simulink library "fdclib3"  (Simulink 2.09)
values from neighbouring files (symbols this model uses):
  GM1 = [cbar b    S    Ix   Iy   Iz   Jxy  Jxz  Jyz  m]    [modbuild.m]

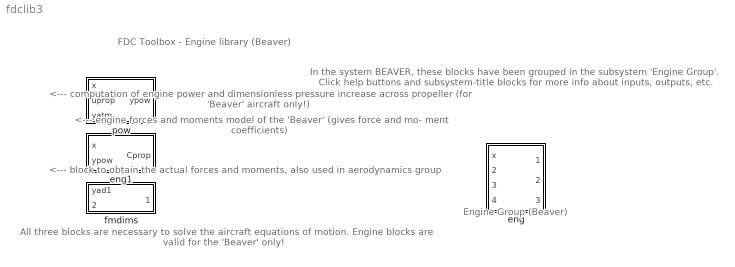
== system fdclib3 ==
  note: FDC Toolbox - Engine library (Beaver)
  note: All three blocks are necessary to solve the aircraft equations
      | of motion. Engine blocks are valid for the 'Beaver' only!
  note: Engine Group
      | (Beaver)
  note: In the system BEAVER, these blocks have
      | been grouped in the subsystem 'Engine Group'.
      | Click help buttons and subsystem-title blocks
      | for more info about inputs, outputs, etc.
  note: <--- block to obtain the actual
      |       forces and moments, also used
      | in aerodynamics group
  note: <--- engine forces and moments model
      | of the 'Beaver' (gives force and mo-
      | ment coefficients)
  note: <--- computation of engine power and
      | dimensionless pressure increase across
      | propeller (for 'Beaver' aircraft only!)
  eng : Subsystem
  eng1 : Subsystem
      mask Type: Engmod
      mask Description: Engine model for the DHC-2 'Beaver'
      mask Help: eval('fdchelp engmod')
      mask Display: disp('Engmod\n(Beaver)')
  fmdims : Subsystem  mask(FMdims){cbar=GM1(1), b=GM1(2), S=GM1(3)}
      mask prompts: cbar "Mean aerodynamic chord [m]:"; b "Wing span [m]:"; S "Wing surface [m^2]:"
      mask help:
      | Calculate forces and moments from
      | dimensionless coefficients.
      mask Help: eval('fdchelp fmdims')
      mask Display: disp('FMdims')
  pow : Subsystem
      mask Type: Power
      mask Description:
      | Engine power and dimensionless
      | pressure increase across propeller
      | (model for DHC-2 'Beaver')
      mask Help: eval('fdchelp power')
      mask Display: disp('Power\n(Beaver)')

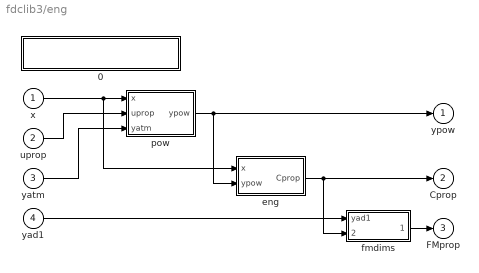
== system fdclib3/eng ==
  x : Inport  Port=1  PortWidth=-1  SampleTime=-1
  uprop : Inport  Port=2  PortWidth=-1  SampleTime=-1
  yatm : Inport  Port=3  PortWidth=-1  SampleTime=-1
  yad1 : Inport  Port=4  PortWidth=-1  SampleTime=-1
  0 : Subsystem
      settings: OpenFcn=fdchelp enggrp
      mask Display: disp('ENGINE GROUP (level 3)\nM.O. Rauw')
  eng : Subsystem
      mask Type: Engmod
      mask Description: Engine model for the DHC-2 'Beaver'
      mask Help: eval('fdchelp engmod')
      mask Display: disp('Engmod\n(Beaver)')
  fmdims : Subsystem  mask(FMdims){cbar=GM1(1), b=GM1(2), S=GM1(3)}
      mask prompts: cbar "Mean aerodynamic chord [m]:"; b "Wing span [m]:"; S "Wing surface [m^2]:"
      mask help:
      | Calculate forces and moments from
      | dimensionless coefficients.
      mask Help: eval('fdchelp fmdims')
      mask Display: disp('FMdims')
  pow : Subsystem
      mask Type: Power
      mask Description:
      | Engine power and dimensionless
      | pressure increase across propeller
      | (model for DHC-2 'Beaver')
      mask Help: eval('fdchelp power')
      mask Display: disp('Power\n(Beaver)')
  ypow : Outport  Port=1  InitialOutput=0
  Cprop : Outport  Port=2  InitialOutput=0
  FMprop : Outport  Port=3  InitialOutput=0
  wires:
  yatm/1 -> pow/3(yatm)
  x/1 -> eng/1(x), pow/1(x)
  yad1/1 -> fmdims/1(yad1)
  eng/1(Cprop) -> fmdims/2(Force / moment coefficients), Cprop/1
  fmdims/1(Forces and moments) -> FMprop/1
  uprop/1 -> pow/2(uprop)
  pow/1(ypow) -> eng/2(ypow), ypow/1

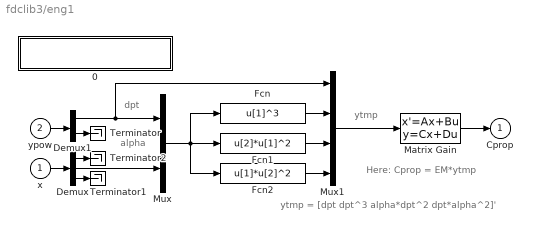
== system fdclib3/eng1 ==
  note: ytmp
  note: alpha
  note: dpt
  note: ytmp = [dpt dpt^3 alpha*dpt^2 dpt*alpha^2]'
  note: Here: Cprop = EM*ytmp
  x : Inport  Port=1  PortWidth=-1  SampleTime=-1
  ypow : Inport  Port=2  PortWidth=-1  SampleTime=-1
  0 : Subsystem
      settings: OpenFcn=fdchelp engmod
      mask Display: disp('ENGMOD\nM.O. Rauw, Dec. 1996')
  Demux : Demux  Outputs=[1 1 10]
  Demux1 : Demux  Outputs=2
  Fcn : Fcn  Expr=u[1]^3
  Fcn1 : Fcn  Expr=u[2]*u[1]^2
  Fcn2 : Fcn  Expr=u[1]*u[2]^2
  Matrix Gain : StateSpace  A=A  B=B  C=C  D=D  X0=0  mask(Matrix Gain){@1=EM}
      mask prompts: @1 "Gain matrix:"
      mask help: Matrix Gain
      mask init:
      | A = []; B = []; C = []; D = @1;
      mask Help: This block implements an matrix gain.\nThe matrix dimensions must be in accordance\nwith the dimension of the inputvector.
      mask Display: disp('y = A*u')
  Mux : Mux  Inputs=2
  Mux1 : Mux  Inputs=4
  Terminator : Terminator
  Terminator1 : Terminator
  Terminator2 : Terminator
  Cprop : Outport  Port=1  InitialOutput=0
  wires:
  Fcn2/1 -> Mux1/4
  Fcn1/1 -> Mux1/3
  Fcn/1 -> Mux1/2
  Demux1/1 -> Mux1/1, Mux/1
  Mux/1 -> Fcn2/1, Fcn/1, Fcn1/1
  Demux/2 -> Mux/2
  ypow/1 -> Demux1/1
  x/1 -> Demux/1
  Mux1/1 -> Matrix Gain/1
  Matrix Gain/1 -> Cprop/1
  Demux1/2 -> Terminator/1
  Demux/3 -> Terminator1/1
  Demux/1 -> Terminator2/1

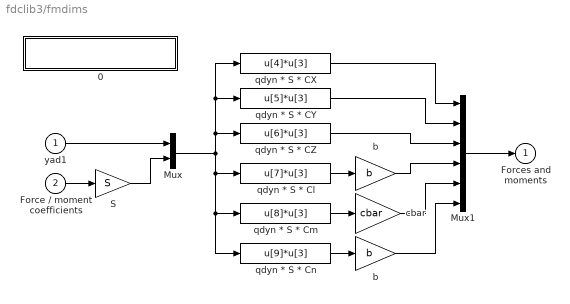
== system fdclib3/fmdims ==
  yad1 : Inport  Port=1  PortWidth=-1  SampleTime=-1
  Force / moment coefficients : Inport  Port=2  PortWidth=-1  SampleTime=-1
  0 : Subsystem
      settings: OpenFcn=fdchelp fmdims
      mask Display: disp('FMDIMS\nM.O. Rauw, October 1997')
  Mux : Mux  Inputs=[3 6]
  Mux1 : Mux  Inputs=6
  S : Gain  Gain=S
  b : Gain  Gain=b
  "b " : Gain  Gain=b
  cbar : Gain  Gain=cbar
  qdyn * S * CX : Fcn  Expr=u[4]*u[3]
  qdyn * S * CY : Fcn  Expr=u[5]*u[3]
  qdyn * S * CZ : Fcn  Expr=u[6]*u[3]
  qdyn * S * Cl : Fcn  Expr=u[7]*u[3]
  qdyn * S * Cm : Fcn  Expr=u[8]*u[3]
  qdyn * S * Cn : Fcn  Expr=u[9]*u[3]
  Forces and moments : Outport  Port=1  InitialOutput=0
  wires:
  b/1 -> Mux1/4
  qdyn * S * CZ/1 -> Mux1/3
  S/1 -> Mux/2
  qdyn * S * CY/1 -> Mux1/2
  qdyn * S * CX/1 -> Mux1/1
  yad1/1 -> Mux/1
  qdyn * S * Cn/1 -> "b "/1
  qdyn * S * Cm/1 -> cbar/1
  qdyn * S * Cl/1 -> b/1
  Mux/1 -> qdyn * S * Cn/1, qdyn * S * Cm/1, qdyn * S * Cl/1, qdyn * S * CY/1, qdyn * S * CX/1, qdyn * S * CZ/1
  Force / moment coefficients/1 -> S/1
  cbar/1 -> Mux1/5
  "b "/1 -> Mux1/6
  Mux1/1 -> Forces and moments/1

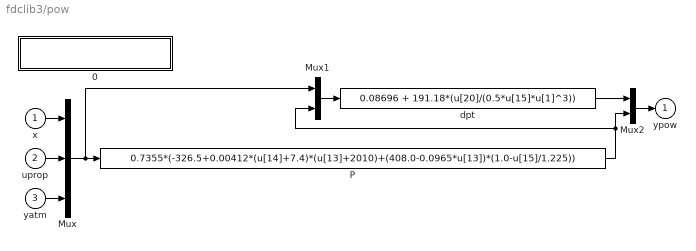
== system fdclib3/pow ==
  x : Inport  Port=1  PortWidth=-1  SampleTime=-1
  uprop : Inport  Port=2  PortWidth=-1  SampleTime=-1
  yatm : Inport  Port=3  PortWidth=-1  SampleTime=-1
  0 : Subsystem
      settings: OpenFcn=fdchelp power
      mask Display: disp('POWER\nM.O. Rauw, October 1997')
  Mux : Mux  Inputs=[12 2 5]
  Mux1 : Mux  Inputs=[19 1]
  Mux2 : Mux  Inputs=2
  P : Fcn  Expr=0.7355*(-326.5+0.00412*(u[14]+7.4)*(u[13]+2010)+(408.0-0.0965*u[13])*(1.0-u[15]/1.225))
  dpt : Fcn  Expr=0.08696 + 191.18*(u[20]/(0.5*u[15]*u[1]^3))
  ypow : Outport  Port=1  InitialOutput=0
  wires:
  Mux1/1 -> dpt/1
  P/1 -> Mux1/2, Mux2/2
  Mux/1 -> Mux1/1, P/1
  x/1 -> Mux/1
  uprop/1 -> Mux/2
  yatm/1 -> Mux/3
  dpt/1 -> Mux2/1
  Mux2/1 -> ypow/1

== system fdclib3/eng/0 ==

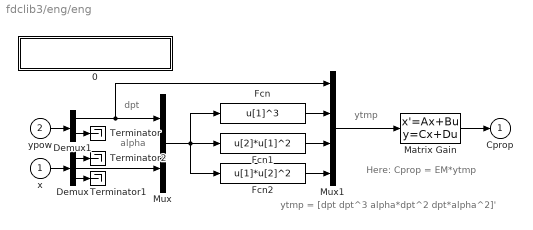
== system fdclib3/eng/eng ==
  note: ytmp
  note: alpha
  note: dpt
  note: ytmp = [dpt dpt^3 alpha*dpt^2 dpt*alpha^2]'
  note: Here: Cprop = EM*ytmp
  x : Inport  Port=1  PortWidth=-1  SampleTime=-1
  ypow : Inport  Port=2  PortWidth=-1  SampleTime=-1
  0 : Subsystem
      settings: OpenFcn=fdchelp engmod
      mask Display: disp('ENGMOD\nM.O. Rauw, Dec. 1996')
  Demux : Demux  Outputs=[1 1 10]
  Demux1 : Demux  Outputs=2
  Fcn : Fcn  Expr=u[1]^3
  Fcn1 : Fcn  Expr=u[2]*u[1]^2
  Fcn2 : Fcn  Expr=u[1]*u[2]^2
  Matrix Gain : StateSpace  A=A  B=B  C=C  D=D  X0=0  mask(Matrix Gain){@1=EM}
      mask prompts: @1 "Gain matrix:"
      mask help: Matrix Gain
      mask init:
      | A = []; B = []; C = []; D = @1;
      mask Help: This block implements an matrix gain.\nThe matrix dimensions must be in accordance\nwith the dimension of the inputvector.
      mask Display: disp('y = A*u')
  Mux : Mux  Inputs=2
  Mux1 : Mux  Inputs=4
  Terminator : Terminator
  Terminator1 : Terminator
  Terminator2 : Terminator
  Cprop : Outport  Port=1  InitialOutput=0
  wires:
  Fcn2/1 -> Mux1/4
  Fcn1/1 -> Mux1/3
  Fcn/1 -> Mux1/2
  Demux1/1 -> Mux1/1, Mux/1
  Mux/1 -> Fcn2/1, Fcn/1, Fcn1/1
  Demux/2 -> Mux/2
  ypow/1 -> Demux1/1
  x/1 -> Demux/1
  Mux1/1 -> Matrix Gain/1
  Matrix Gain/1 -> Cprop/1
  Demux1/2 -> Terminator/1
  Demux/3 -> Terminator1/1
  Demux/1 -> Terminator2/1

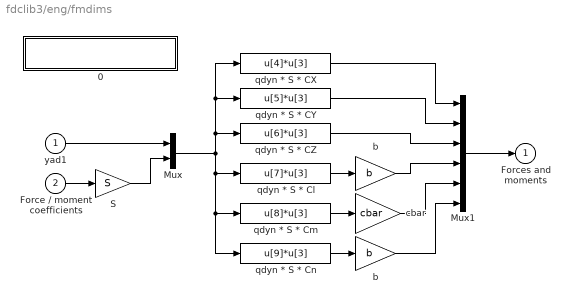
== system fdclib3/eng/fmdims ==
  yad1 : Inport  Port=1  PortWidth=-1  SampleTime=-1
  Force / moment coefficients : Inport  Port=2  PortWidth=-1  SampleTime=-1
  0 : Subsystem
      settings: OpenFcn=fdchelp fmdims
      mask Display: disp('FMDIMS\nM.O. Rauw, October 1997')
  Mux : Mux  Inputs=[3 6]
  Mux1 : Mux  Inputs=6
  S : Gain  Gain=S
  b : Gain  Gain=b
  "b " : Gain  Gain=b
  cbar : Gain  Gain=cbar
  qdyn * S * CX : Fcn  Expr=u[4]*u[3]
  qdyn * S * CY : Fcn  Expr=u[5]*u[3]
  qdyn * S * CZ : Fcn  Expr=u[6]*u[3]
  qdyn * S * Cl : Fcn  Expr=u[7]*u[3]
  qdyn * S * Cm : Fcn  Expr=u[8]*u[3]
  qdyn * S * Cn : Fcn  Expr=u[9]*u[3]
  Forces and moments : Outport  Port=1  InitialOutput=0
  wires:
  b/1 -> Mux1/4
  qdyn * S * CZ/1 -> Mux1/3
  S/1 -> Mux/2
  qdyn * S * CY/1 -> Mux1/2
  qdyn * S * CX/1 -> Mux1/1
  yad1/1 -> Mux/1
  qdyn * S * Cn/1 -> "b "/1
  qdyn * S * Cm/1 -> cbar/1
  qdyn * S * Cl/1 -> b/1
  Mux/1 -> qdyn * S * Cn/1, qdyn * S * Cm/1, qdyn * S * Cl/1, qdyn * S * CY/1, qdyn * S * CX/1, qdyn * S * CZ/1
  Force / moment coefficients/1 -> S/1
  cbar/1 -> Mux1/5
  "b "/1 -> Mux1/6
  Mux1/1 -> Forces and moments/1

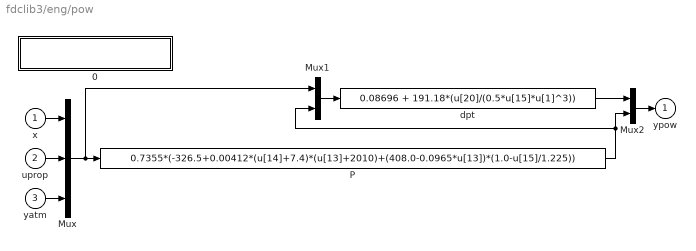
== system fdclib3/eng/pow ==
  x : Inport  Port=1  PortWidth=-1  SampleTime=-1
  uprop : Inport  Port=2  PortWidth=-1  SampleTime=-1
  yatm : Inport  Port=3  PortWidth=-1  SampleTime=-1
  0 : Subsystem
      settings: OpenFcn=fdchelp power
      mask Display: disp('POWER\nM.O. Rauw, October 1997')
  Mux : Mux  Inputs=[12 2 5]
  Mux1 : Mux  Inputs=[19 1]
  Mux2 : Mux  Inputs=2
  P : Fcn  Expr=0.7355*(-326.5+0.00412*(u[14]+7.4)*(u[13]+2010)+(408.0-0.0965*u[13])*(1.0-u[15]/1.225))
  dpt : Fcn  Expr=0.08696 + 191.18*(u[20]/(0.5*u[15]*u[1]^3))
  ypow : Outport  Port=1  InitialOutput=0
  wires:
  Mux1/1 -> dpt/1
  P/1 -> Mux1/2, Mux2/2
  Mux/1 -> Mux1/1, P/1
  x/1 -> Mux/1
  uprop/1 -> Mux/2
  yatm/1 -> Mux/3
  dpt/1 -> Mux2/1
  Mux2/1 -> ypow/1

== system fdclib3/eng1/0 ==

== system fdclib3/fmdims/0 ==

== system fdclib3/pow/0 ==

== system fdclib3/eng/eng/0 ==

== system fdclib3/eng/fmdims/0 ==

== system fdclib3/eng/pow/0 ==
